simulink model "robot_model"  (Simulink 8.9)
settings: Solver=ode45  StartTime=0.0  StopTime=10.0  RelTol=1e-3  EnableMultiTasking=on
undefined symbols (not defined in the file): psi0, u0, UAV_Dynamics, UAV_with_lowlevelcontrol, vx_disturb, vy_disturb, w0, w_max, w_min, x0, y0
settings Model: Creator=user  LastModifiedBy=edward
settings OptimizationCC: ExpressionDepthLimit=2147483647  InitFltsAndDblsToZero=on
settings DebuggingCC: SolverPrmCheckMsg=warning  StrictBusMsg=Warning
settings GRTTargetCC: GeneratePreprocessorConditionals=Use local settings

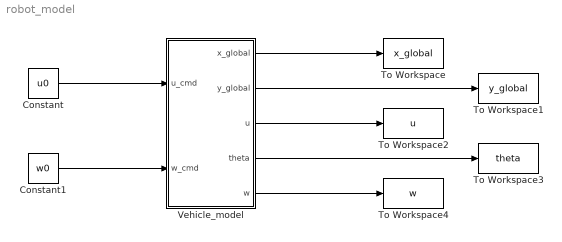
== system robot_model ==
  Constant : Constant  Value=u0
  Constant1 : Constant  Value=w0
  To Workspace : ToWorkspace  VariableName=x_global  SampleTime=-1
  To Workspace1 : ToWorkspace  VariableName=y_global  SampleTime=-1
  To Workspace2 : ToWorkspace  VariableName=u  SampleTime=-1
  To Workspace3 : ToWorkspace  VariableName=theta  SampleTime=-1
  To Workspace4 : ToWorkspace  VariableName=w  SampleTime=-1
  Vehicle_model : Subsystem  AncestorBlock=UAV_Dynamics/UAV_with_lowlevelcontrol
  wires:
  Constant/1 -> Vehicle_model/1(u_cmd)
  Constant1/1 -> Vehicle_model/2(w_cmd)
  Vehicle_model/1(x_global) -> To Workspace/1
  Vehicle_model/2(y_global) -> To Workspace1/1
  Vehicle_model/3(u) -> To Workspace2/1
  Vehicle_model/4(theta) -> To Workspace3/1
  Vehicle_model/5(w) -> To Workspace4/1

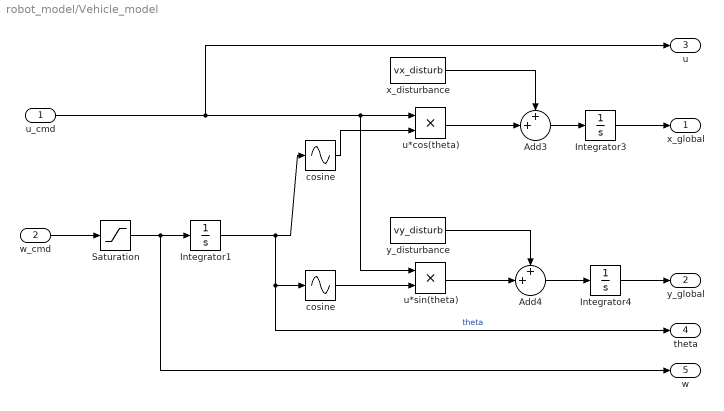
== system robot_model/Vehicle_model ==
  u_cmd : Inport
  w_cmd : Inport  Port=2
  Add3 : Sum  Inputs=++|
  Add4 : Sum  Inputs=++|
  Integrator1 : Integrator  InitialCondition=psi0
  Integrator3 : Integrator  InitialCondition=x0
  Integrator4 : Integrator  InitialCondition=y0
  Saturation : Saturate  UpperLimit=w_max  LowerLimit=w_min
  cosine : Sin  TimeSource=Use external signal  Phase=pi/2  SampleTime=0
  "cosine  " : Sin  TimeSource=Use external signal  SampleTime=0
  u*cos(theta) : Product  RndMeth=Zero
  u*sin(theta) : Product  RndMeth=Zero
  x_disturbance : Constant  Value=vx_disturb
  y_disturbance : Constant  Value=vy_disturb
  x_global : Outport
  y_global : Outport  Port=2
  u : Outport  Port=3
  theta : Outport  Port=4
  w : Outport  Port=5
  wires:
  Add4/1 -> Integrator4/1
  u*sin(theta)/1 -> Add4/2
  y_disturbance/1 -> Add4/1
  Add3/1 -> Integrator3/1
  u*cos(theta)/1 -> Add3/2
  x_disturbance/1 -> Add3/1
  Integrator4/1 -> y_global/1
  Integrator3/1 -> x_global/1
  Saturation/1 -> w/1, Integrator1/1
  Integrator1/1 -> cosine/1, "cosine  "/1, theta/1  "theta"
  cosine/1 -> u*cos(theta)/2
  "cosine  "/1 -> u*sin(theta)/2
  u_cmd/1 -> u*cos(theta)/1, u*sin(theta)/1, u/1
  w_cmd/1 -> Saturation/1
